simulink model "S3"  (R2023b)
settings: Solver=FixedStepAuto  StartTime=0.0  StopTime=Time  FixedStep=Step_T  RelTol=1e-3
InitFcn:
  | run("P_sim.m")
values from neighbouring files (symbols this model uses):
  x_1_0 = 0.5    [P_sim.m]
  x_2_0 = -0.5    [P_sim.m]
settings Model: Creator=admin  LastModifiedBy=admin

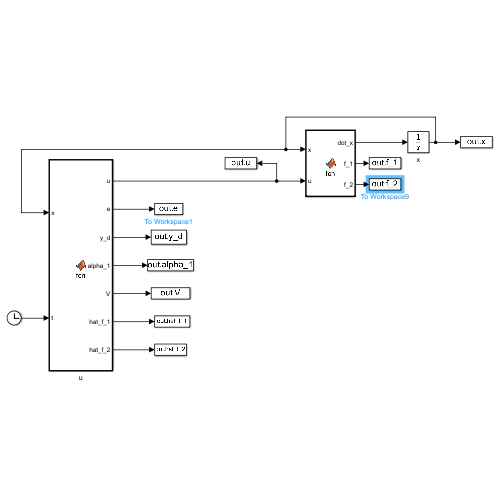
[thumbnail: Simulink's stored preview of the top-level diagram]
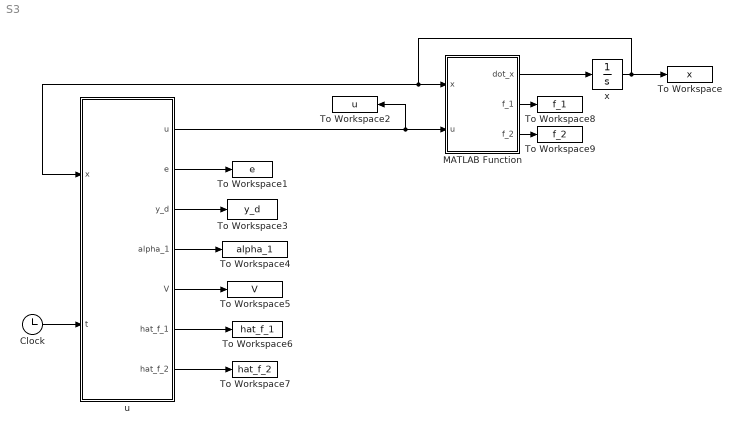
== system S3 ==
  Clock : Clock
  MATLAB Function : MATLAB Function  TreatAsAtomicUnit=on
  To Workspace : ToWorkspace  VariableName=x  SaveFormat=Timeseries  SampleTime=-1
  To Workspace1 : ToWorkspace  VariableName=e  SaveFormat=Timeseries  SampleTime=-1
  To Workspace2 : ToWorkspace  VariableName=u  SaveFormat=Timeseries  SampleTime=-1
  To Workspace3 : ToWorkspace  VariableName=y_d  SaveFormat=Timeseries  SampleTime=-1
  To Workspace4 : ToWorkspace  VariableName=alpha_1  SaveFormat=Timeseries  SampleTime=-1
  To Workspace5 : ToWorkspace  VariableName=V  SaveFormat=Timeseries  SampleTime=-1
  To Workspace6 : ToWorkspace  VariableName=hat_f_1  SaveFormat=Timeseries  SampleTime=-1
  To Workspace7 : ToWorkspace  VariableName=hat_f_2  SaveFormat=Timeseries  SampleTime=-1
  To Workspace8 : ToWorkspace  VariableName=f_1  SaveFormat=Timeseries  SampleTime=-1
  To Workspace9 : ToWorkspace  VariableName=f_2  SaveFormat=Timeseries  SampleTime=-1
  u : MATLAB Function  TreatAsAtomicUnit=on
  x : Integrator  InitialCondition=[x_1_0;x_2_0]
  wires:
  MATLAB Function/1(dot_x) -> x/1
  x/1 -> To Workspace/1, u/1(x), MATLAB Function/1(x)
  u/1(u) -> To Workspace2/1, MATLAB Function/2(u)
  u/2(e) -> To Workspace1/1
  u/3(y_d) -> To Workspace3/1
  u/4(alpha_1) -> To Workspace4/1
  u/5(V) -> To Workspace5/1
  Clock/1 -> u/2(t)
  u/6(hat_f_1) -> To Workspace6/1
  u/7(hat_f_2) -> To Workspace7/1
  MATLAB Function/2(f_1) -> To Workspace8/1
  MATLAB Function/3(f_2) -> To Workspace9/1

== matlab function S3/u ==
  data: x input; t input; u output; e output; pam parameter; y_d output; alpha_1 output; V output; hat_f_1 output; hat_f_2 output
function [u,e,y_d,alpha_1,V,hat_f_1,hat_f_2]  = fcn(x,t,pam)

y_d = sin(t);
dot_y_d = cos(t);
ddot_y_d = -sin(t);

x_1 = x(1);
x_2 = x(2);

z_1 = [x_1;x_1^2];
z_2 = [x_1;x_2;x_1*x_2;x_1^2;x_2^2];

dot_x_1 = x_2-2*x_1;

%% 第一阶
e_1 = x_1 - y_d;
alpha_1 = -pam.lambda_1*e_1-pam.hat_theta_1'*z_1+dot_y_d;
 
%% 第二阶
e_2 = x_2 - alpha_1;
dot_alpha_1 = -pam.lambda_1*(dot_x_1-dot_y_d)+2*dot_x_1+ddot_y_d;
u = -pam.lambda_2*e_2-pam.hat_theta_2'*z_2+dot_alpha_1;

e = [e_1;e_2];

V = e'*pam.S*e;

hat_f_1 = pam.hat_theta_1'*z_1;
hat_f_2 = pam.hat_theta_2'*z_2;

== matlab function S3/MATLAB Function ==
  data: x input; dot_x output; u input; f_1 output; f_2 output
function [dot_x,f_1,f_2]  = fcn(x,u)

x_1 = x(1);
x_2 = x(2);

f_1 = -2*x_1;
f_2 = +3*x_1-x_1*x_2+x_2^2;

dot_x_1 = x_2+f_1;
dot_x_2 = u+f_2;

dot_x = [dot_x_1;dot_x_2];
